simulink model "mech_flexible_cantilever_multiaxis"  (Simulink 7.1)
settings: Solver=ode23tb  StartTime=0.0  StopTime=5  RelTol=1e-2
InitFcn:
  | %-----------------------------------------
  | % Defined in the block mask now. I have left it here because it can be
  | % used as a starting point of describing a material data file format
  | %-----------------------------------------
  | fBeamElement.material = 'Mild Steel';
  | 
  | % Beam element density (Kg/m^3)
  | fBeamElement.density = 7800;
  | 
  | % Length and Width
  | fBeamElement.LengX = 1E-2;
  | fBeamElement.LengY = 1E-2;
  | 
  | % Beam element area of cross-section (m^2)
  | fBeamElement.crossArea = fBeamElement.LengX * fBeamElement.LengY;
  | 
  | % Beam element length (m)
  | fBeamElement.length = 0.2;
  | 
  | % Length of CG vector along length of beam (m)
  | fBeamElement.cgLeng = fBeamElement.length/2;
  | 
  | % Beam element direction (along X direction it is [1 0 0])
  | fBeamElement.beamDir = [1 0 0];
  | 
  | % Beam element Mass Moment of Inertia (Kg/m^2)
  | fBeamElement.Inertia = [0.5 0 0;0 6.3 0;0 0 6.3]*8E-5;
  | 
  | % Beam element Youngs Modulus (N/m^2)
  | fBeamElement.youngsM = 210E9;
  | 
  | % Beam element Shear Modulus (N/m^2)
  | fBeamElement.shearM = 26E9;
  | 
  | % Beam element Area Moment of Inertia along the direction of bending (m^4)
  | fBeamElement.Ixx = fBeamElement.LengX * fBeamElement.LengY^3/12;
  | 
  | % Beam element Area Moment of Inertia normal to the direction of
  | % bending (m^4)
  | fBeamElement.Iyy = fBeamElement.LengY * fBeamElement.LengX^3/12;
  | 
  | % Damping Coeff
  | fBeamElement.matDamping = 1.8;
  | %-----------------------------------------
undefined symbols (not defined in the file or in its folder): sigbuilder_block
libraries: mblibv1 x5, mech_flexible_element_lib x5
Description:
  | Multiaxis Flexible Cantilever
  | 
  | This flexible multiaxis cantilever can twist about its cross-section and elongate about its length. For a brief time, the cantilever is subject to a load modeling a hammer. The cantilever is also subject to its own weight in gravity.
settings Model: Creator=arnav  LastModifiedBy=batserve  ExtModeAutoUpdateStatusClock=off
settings SolverCC: MaxOrder=3
settings DataIOCC: OutputOption=SpecifiedOutputTimes  OutputTimes=linspace(0,5,500)
settings DebuggingCC: SaveWithParameterizedLinksMsg=none  SignalResolutionControl=TryResolveAllWithWarning  SolverPrmCheckMsg=none  MultiTaskDSMMsg=warning  MultiTaskCondExecSysMsg=none  SigSpecEnsureSampleTimeMsg=none  StrictBusMsg=None
settings HardwareCC: TargetBitPerLong=64  TargetEndianess=LittleEndian  TargetWordSize=64  TargetHWDeviceType=MATLAB Host  ProdEqTarget=off
settings RTWCC: SystemTargetFile=rsim.tlc  TemplateMakefile=rsim_default_tmf  Description=Rapid Simulation Target  ProcessScript=rsim_make_rtw_hook  IncludeERTFirstTime=on
settings RSimTargetCC: TargetFcnLib=ansi_tfl_tmw.mat  TargetFunctionLibrary=ANSI_C  IsPILTarget=off  EnableShiftOperators=on  PortableWordSizes=off
settings SimMechanicsCC: VisConfigFile=mech_flexible_cantilever_multiaxis.mat

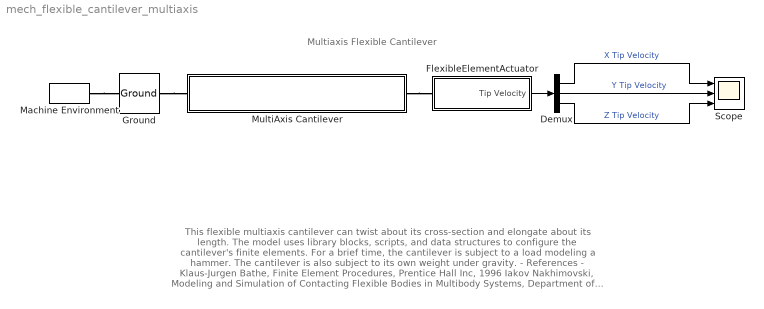
== system mech_flexible_cantilever_multiaxis ==
  note: This flexible multiaxis cantilever can twist about its cross-section and
      | elongate about its length.  The model uses library blocks, scripts, and
      | data structures to configure the cantilever's finite elements.
      |
      | For a brief time, the cantilever is subject to a load modeling a hammer.
      | The cantilever is also subject to its own weight under gravity.
      |
      |  - References -
      |
      | Klaus-Jurgen Bathe, Finite Element Procedures, Prentice Hall Inc, 1996
      |
      | Iakov Nakhimovski, Modeling and Simulation of Contacting Flexible Bodies in Multibody Systems,
      | Department of Computer and Information Science,
      | Lingoping University, Sweden, 2002, Thesis No 989
  note: Multiaxis Flexible Cantilever
  Demux : Demux  Outputs=3
  FlexibleElementActuator : Subsystem
  Ground : mblibv1/Bodies/Ground  DialogController=MECH.DynMechDlgSource  SystemSampleTime=-1  LeftPortType=env  RightPortType=workingframe  PhysicalDomain=Mechanical  DialogClass=GroundBlock  CoordPosition=[0 0 0]  CoordPositionUnits=m  StateVectorMgrId=-1  MachineId=[0 0]  ShowEnvPort=on
  Machine Environment : mblibv1/Bodies/Machine Environment  Tag=Factory ground  DialogController=MECH.DialogSource  SystemSampleTime=-1  PortType=env  PhysicalDomain=Mechanical  DialogTemplateClass=MECH.MachineEnvironment  SyncWhenCopied=off  Gravity=[0 -9.81 0]  GravityUnits=m/s^2  GravityAsSignal=off  Dimensionality=Auto-detect  AnalysisType=Forward dynamics  LinearAssemblyTolerance=1e-3  LinearAssemblyToleranceUnits=m  AngularAssemblyTolerance=1e-3  AngularAssemblyToleranceUnits=rad  ConstraintSolverType=Stabilizing  ConstraintRelTolerance=1e-4  ConstraintAbsTolerance=1e-4  UseRobustSingularityHandling=off  RedundancyAnalysisToleranceType=Automatically select tolerance  RedundancyAnalysisTolerance=1e-14  StatePerturbationType=Fixed  PerturbationSize=1e-5  VisualizeMachine=on
  MultiAxis Cantilever : Subsystem
  Scope : Scope  NumInputPorts=3
      settings: TimeRange=5  YMin=-5~-4~-4  YMax=15~1~6
  wires:
  Demux/1 -> Scope/1  "X Tip Velocity"
  Demux/2 -> Scope/2  "Y Tip Velocity"
  Demux/3 -> Scope/3  "Z Tip Velocity"
  FlexibleElementActuator/1(Tip Velocity) -> Demux/1
  connections:
  Machine Environment/RConn1 -- Ground/LConn1
  Ground/RConn1 -- MultiAxis Cantilever/LConn1
  MultiAxis Cantilever/RConn1 -- FlexibleElementActuator/LConn1

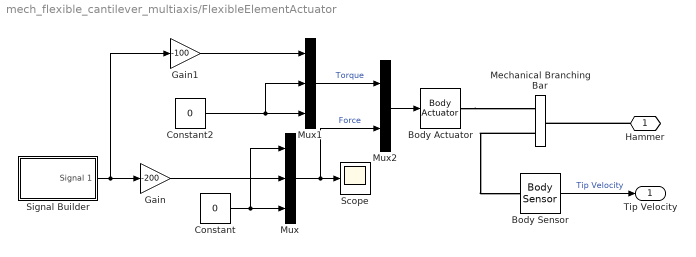
== system mech_flexible_cantilever_multiaxis/FlexibleElementActuator ==
  Body Actuator : mblibv1/Sensors &  Actuators/Body Actuator  DialogController=MECH.DynMechDlgSource  SystemSampleTime=-1  PhysicalDomain=Mechanical  PortType=blob  ActuationStyle=Force  AngleUnits=deg  ArcVelocityUnits=deg/s  ArcAccelerationUnits=deg/s^2  CoordPositionUnits=m  VelocityUnits=m/s  AccelerationUnits=m/s^2  ForceUnits=N  TorqueUnits=N-m  ActiveIO=on  Width=6  DialogClass=MechanicalActuatorBlock  ReferenceFrame=Absolute (World)  Angle=off  CoordPosition=on  Force=on  Torque=on
  Body Sensor : mblibv1/Sensors &  Actuators/Body Sensor  DialogController=MECH.DynMechDlgSource  SystemSampleTime=-1  PhysicalDomain=Mechanical  PortType=blob  Muxed=on  Pose=off  Angle=on  AngleUnits=deg  ArcVelocity=on  ArcVelocityUnits=rad/s  ArcAcceleration=off  ArcAccelerationUnits=deg/s^2  CoordPosition=off  CoordPositionUnits=m  Velocity=off  VelocityUnits=m/s  Acceleration=off  AccelerationUnits=m/s^2  Quaternion=on  QuaternionDT=off  QuaternionDDT=off  QuaternionUnits=off  OutputVector=[ 3 ]  ActiveIO=on  Width=3  DialogClass=MechanicalSensorBlock  ReferenceFrame=Absolute (World)
  Constant : Constant  Value=0  OutDataType=sfix(16)  OutScaling=2^0
  Constant2 : Constant  Value=0  OutDataType=sfix(16)  OutScaling=2^0
  Gain : Gain  Gain=-200  ParameterDataType=sfix(16)  ParameterScaling=2^0  OutDataType=sfix(16)  OutScaling=2^0
  Gain1 : Gain  Gain=-100  ParameterDataType=sfix(16)  ParameterScaling=2^0  OutDataType=sfix(16)  OutScaling=2^0
  Mechanical Branching Bar : mblibv1/Utilities/Mechanical Branching Bar  Orientation=left  DialogController=MECH.DynMechDlgSource  PhysicalDomain=mechanical  SubClassName=Unknown  LeftPortType=blob  RightPortType=blob  LConnTagsString=_newl0  RConnTagsString=SA0|SA1  DialogClass=MechanicalBranchingBarBlock  NumSAPorts=2
  Mux : Mux  Inputs=3
  Mux1 : Mux  Inputs=3
  Mux2 : Mux  Inputs=2
  Scope : Scope
      settings: TimeRange=5  YMin=-200  YMax=0
  Signal Builder : Subsystem  Tag=STV Subsys  LoadFcn=sigbuilder_block('load');  StartFcn=sigbuilder_block('start');  StopFcn=sigbuilder_block('stop');  ClipboardFcn=sigbuilder_block('clipboard');  mask(Sigbuilder block){}
      mask help: Sigbuilder GUI
      mask init:
      | if ~strcmp(get_param(bdroot(gcbh),'SimulationStatus'),'stopped') tuvar = sigbuilder_block('maskInit'); end
      settings: CopyFcn=sigbuilder_block('copy');  DeleteFcn=sigbuilder_block('delete');  ModelCloseFcn=sigbuilder_block('modelClose');  PreSaveFcn=sigbuilder_block('preSave');  NameChangeFcn=sigbuilder_block('namechange');  OpenFcn=sigbuilder_block('open',[31.5 93 550.5 399.75 ]);  CloseFcn=sigbuilder_block('close');
      mask Display: plot(0,0,100,100,[10,10,40,40,10],[80,20,20,80,80],[40,10],[50,50], [40,27,10],[65,72,56],[40,25,25,10],[28,28,43,43]);
  Hammer : PMIOPort  Orientation=left  Port=1  Side=Left
  Tip Velocity : Outport  OutDataType=sfix(16)  OutScaling=2^0
  wires:
  Mux1/1 -> Mux2/1  "Torque"
  Mux2/1 -> Body Actuator/1
  Gain/1 -> Mux/2
  Signal Builder/1(Signal 1) -> Gain/1, Gain1/1
  Body Sensor/1 -> Tip Velocity/1  "Tip Velocity"
  Mux/1 -> Mux2/2, Scope/1  "Force"
  Constant/1 -> Mux/3, Mux/1
  Constant2/1 -> Mux1/3, Mux1/2
  Gain1/1 -> Mux1/1
  connections:
  Hammer/RConn1 -- Mechanical Branching Bar/LConn1
  Body Actuator/RConn1 -- Mechanical Branching Bar/RConn1
  Mechanical Branching Bar/RConn2 -- Body Sensor/LConn1

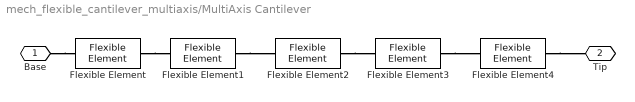
== system mech_flexible_cantilever_multiaxis/MultiAxis Cantilever ==
  Flexible Element{,1..4} (5 alike) : mech_flexible_element_lib/Flexible Element  SystemSampleTime=-1  material=Mild Steel  density=fBeamElement.density  crossArea=fBeamElement.crossArea  length=fBeamElement.length  cgLeng=fBeamElement.cgLeng  beamDir=fBeamElement.beamDir  Inertia=fBeamElement.Inertia  youngsM=fBeamElement.youngsM  shearM=fBeamElement.shearM  Ixx=fBeamElement.Ixx  Iyy=fBeamElement.Iyy  matDamping=fBeamElement.matDamping
  Base : PMIOPort  Port=1  Side=Left
  Tip : PMIOPort  Orientation=left  Port=2  Side=Right
  connections:
  Base/RConn1 -- Flexible Element/LConn1
  Flexible Element/RConn1 -- Flexible Element1/LConn1
  Flexible Element1/RConn1 -- Flexible Element2/LConn1
  Flexible Element2/RConn1 -- Flexible Element3/LConn1
  Flexible Element3/RConn1 -- Flexible Element4/LConn1
  Flexible Element4/RConn1 -- Tip/RConn1

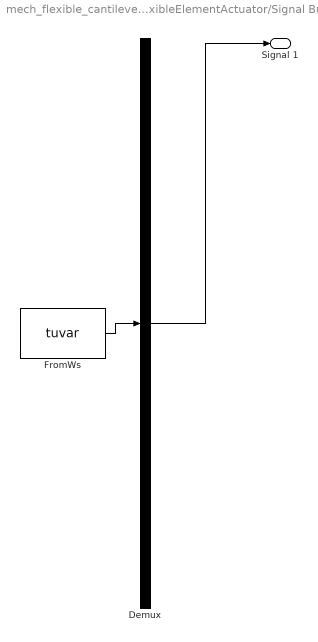
== system mech_flexible_cantilever_multiaxis/FlexibleElementActuator/Signal Builder ==
  Demux : Demux  Tag=STV Demux  Outputs=1
  FromWs : FromWorkspace  Tag=STV FromWs  VariableName=tuvar  SampleTime=0  SigBuilderData=DataTag0  VnvData=DataTag1
      SigBuilderData=|
      | channels.label = 'Signal 1'
      | channels.allXData = {[0 0.1 1 1.5 1.7 10]}
      | channels.allYData = {[0 0 1 1 0 0]}
      | common.afterFinalStr = 'Extrapolate'
      | common.sampleTime = 0
      | dataSet.timeRange = [0 10]
      | dataSet.name = 'Group 1'
  Signal 1 : Outport  Tag=STV Outport  OutDataType=sfix(16)  OutScaling=2^0
  wires:
  FromWs/1 -> Demux/1
  Demux/1 -> Signal 1/1
